simulink model "sistema_term"  (R2021b)
settings: Solver=FixedStepDiscrete  StartTime=0.0  StopTime=90  FixedStep=Tint  RelTol=1e-3
InitFcn:
  | init_fcn
values from neighbouring files (symbols this model uses):
  C_load = 5e-2    (= 0.05)    [init_fcn.m]
  C_V = c_v * ro_air * volume_room    (= 220.63309632)    [init_fcn.m]
  K_cond = Window_area * k_glass / esp    (= 158.4)    [init_fcn.m]
  L_s = 5e-3    (= 0.005)    [init_fcn.m]
  shift = (180/3)/360 * Ts    (= 8.33333333333e-05)    [init_fcn.m]
  T_ext = 15    [init_fcn.m]
  Tint = 5e-5    (= 5e-05)    [init_fcn.m]
  Ts = 0.0005    [init_fcn.m]
  V_H4 = 300    [init_fcn.m]
  V_source = 230 * sqrt(2)    [init_fcn.m]
undefined symbols (not defined in the file or in its folder): DiscIntNeverNeededParam
libraries: spsIGBTDiodeLib x5, spsSeriesRLCBranchLib x4, spsCurrentMeasurementLib x4, spsVoltageMeasurementLib x4, slpidlib x3, simulink x3, spsACVoltageSourceLib x1, spsDiodeLib x1, spsParallelRLCBranchLib x1, spspowerguiLib x1
settings Model: Creator=david  LastModifiedBy=david

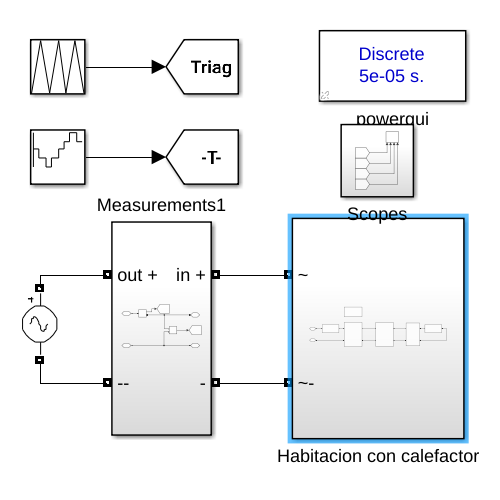
[thumbnail: Simulink's stored preview of the top-level diagram]
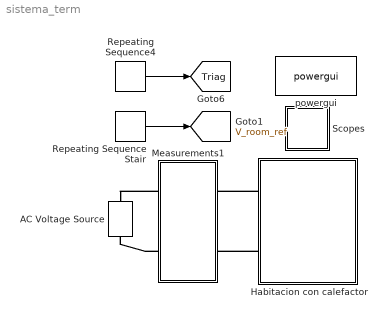
== system sistema_term ==
  AC Voltage Source : spsACVoltageSourceLib/AC Voltage Source  Amplitude=V_source  Phase=0  Frequency=50  SampleTime=0  Measurements=None  BusType=swing  Pref=10e3  Qref=0  Qmin=-inf  Qmax=+inf
  Habitacion con calefactor : Subsystem
  Measurements1 : Subsystem
  Repeating Sequence Stair : simulink/Sources/Repeating Sequence Stair  OutValues=[300 200 100 200 300 400 500 400].'  tsamp=10  OutMin=[]  OutMax=[]  OutDataTypeStr=double  OutputDataTypeScalingMode=double  OutDataType=fixdt(0,8)  ConRadixGroup=Best Precision: Vector-wise  OutScaling=2^-12
  Repeating Sequence4 : simulink/Sources/Repeating Sequence  rep_seq_t=[0 Ts/2 Ts]  rep_seq_y=[-1 1 -1]
  Scopes : Subsystem
  powergui : spspowerguiLib/powergui  Priority=1  SimulationMode=Discrete  SampleTime=Tint  frequency=60  Iterations=50  frequencyindice=0  Pbase=100e6  ErrMax=1e-4  UnitsV=kV  UnitsW=MW  buscounter=0  FunctionMessages=off  echomessages=off  EnableUseOfTLC=off  CurrentSourceSwitches=off  DisableSnubberDevices=off  DisableRonSwitches=off  DisableVfSwitches=off  DisplayEquations=off  AutomaticDiscreteSolvers=off  SolverType=Tustin/Backward Euler (TBE)  Interpol=off  ExternalGateDelay=off  methode=off  Ts=100  x0status=blocks  SPID=on  SwTol=0  HookPort=off  NonlinearTolerance=1e-4  nMaxIteration=100  ContinueOnMaxIteration=off  RestoreLinks=warning  ResistiveCurrentMeasurement=off  Frange=[0:2:500]  Ylog=off  Xlog=on  ShowGrid=off  save=off  variable=ZData  structure=0  ZoomFFT=off  StartTime=0.0  cycles=1  DisplayStyle=1  fundamental=60  FreqAxis=off  MaxFrequency=1000  frequencyindicesteady=1  RmsSteady=1  display=off
  tag scope: Triag=global, V_room_ref=global
  wires:
  Repeating Sequence4/1 -> [Triag]
  Repeating Sequence Stair/1 -> [V_room_ref]
  connections:
  Measurements1/RConn1 -- AC Voltage Source/RConn1
  Measurements1/RConn2 -- AC Voltage Source/LConn1
  Habitacion con calefactor/LConn1 -- Measurements1/LConn1
  Habitacion con calefactor/LConn2 -- Measurements1/LConn2

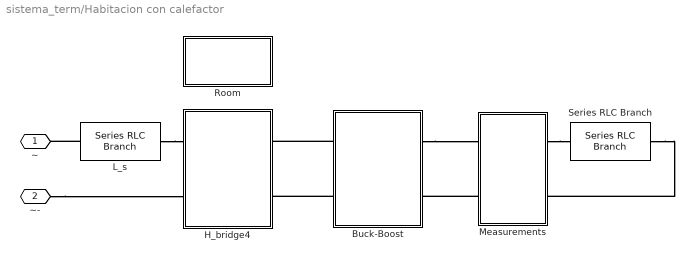
== system sistema_term/Habitacion con calefactor ==
  Buck-Boost : Subsystem
  H_bridge4 : Subsystem
  L_s : spsSeriesRLCBranchLib/Series RLC Branch  LConnTagsString=__new0  RConnTagsString=__new0  BranchType=L  Resistance=1  Inductance=L_s  SetiL0=off  InitialCurrent=0  Capacitance=1e-6  Setx0=off  InitialVoltage=0  Measurements=None
  Measurements : Subsystem
  Room : Subsystem
  Series RLC Branch : spsSeriesRLCBranchLib/Series RLC Branch  LConnTagsString=__new0  RConnTagsString=__new0  BranchType=R  Resistance=100  Inductance=1e-3  SetiL0=off  InitialCurrent=0  Capacitance=1e-6  Setx0=off  InitialVoltage=0  Measurements=None
  ~ : PMIOPort  Side=Left
  ~- : PMIOPort  Port=2  Side=Left
  connections:
  ~-/RConn1 -- H_bridge4/RConn2
  L_s/LConn1 -- H_bridge4/RConn1
  L_s/RConn1 -- ~/RConn1
  Measurements/RConn1 -- Series RLC Branch/LConn1
  Series RLC Branch/RConn1 -- Measurements/RConn2
  Buck-Boost/RConn1 -- Measurements/LConn1
  Measurements/LConn2 -- Buck-Boost/RConn2
  Buck-Boost/LConn2 -- H_bridge4/LConn2
  Buck-Boost/LConn1 -- H_bridge4/LConn1

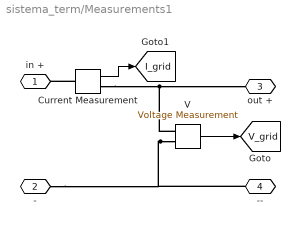
== system sistema_term/Measurements1 ==
  Current Measurement : spsCurrentMeasurementLib/Current Measurement  PhasorSimulation=off  OutputType=Complex  PSBequivalent=0
  V : spsVoltageMeasurementLib/Voltage Measurement  PhasorSimulation=off  OutputType=Complex  PSBequivalent=0
  in + : PMIOPort  Side=Left
  - : PMIOPort  Port=2  Side=Left
  out + : PMIOPort  Port=3  Side=Right
  -- : PMIOPort  Port=4  Side=Right
  tag scope: I_grid=global, V_grid=global
  wires:
  V/1 -> [V_grid]
  Current Measurement/1 -> [I_grid]
  connections:
  V/LConn2 -- --/RConn1 -- -/RConn1
  V/LConn1 -- Current Measurement/RConn1 -- out +/RConn1
  Current Measurement/LConn1 -- in +/RConn1

== system sistema_term/Scopes ==
  Scope : Scope  NumInputPorts=4
  wires:
  [V_room_ref] -> Scope/2
  [T_room] -> Scope/1
  [V_room] -> Scope/4
  [P_room] -> Scope/3

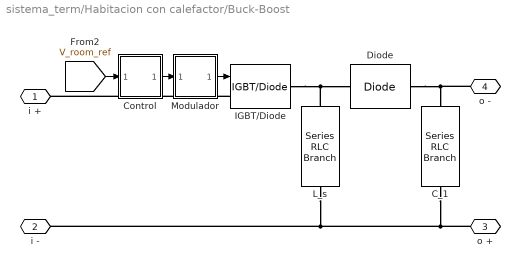
== system sistema_term/Habitacion con calefactor/Buck-Boost ==
  C_1 : spsSeriesRLCBranchLib/Series RLC Branch  LConnTagsString=__new0  RConnTagsString=__new0  BranchType=C  Resistance=1  Inductance=L_s/2  SetiL0=off  InitialCurrent=0  Capacitance=C_load/4  Setx0=on  InitialVoltage=300  Measurements=None
  Control : Subsystem
  Diode : spsDiodeLib/Diode  Ron=1e-3  Lon=0  Vf=0.8  IC=0  UseSnubber=0  Rs=1e3  Cs=250e-9  Measurements=off
  IGBT/Diode : spsIGBTDiodeLib/IGBT//Diode  Ron=1e-3  Rs=1e5  Cs=inf  Measurements=off
  L_s : spsSeriesRLCBranchLib/Series RLC Branch  LConnTagsString=__new0  RConnTagsString=__new0  BranchType=L  Resistance=1  Inductance=L_s * 12  SetiL0=off  InitialCurrent=0  Capacitance=1e-6  Setx0=off  InitialVoltage=0  Measurements=None
  Modulador : Subsystem
  i + : PMIOPort  Side=Left
  i - : PMIOPort  Port=2  Side=Left
  o + : PMIOPort  Port=3  Side=Right
  o - : PMIOPort  Port=4  Side=Right
  wires:
  Control/1(Out1) -> Modulador/1(In1)
  Modulador/1(Out1) -> IGBT/Diode/1
  [V_room_ref] -> Control/1(In1)
  connections:
  C_1/LConn1 -- L_s/LConn1 -- i -/RConn1 -- o +/RConn1
  L_s/RConn1 -- Diode/RConn1 -- IGBT/Diode/RConn1
  o -/RConn1 -- Diode/LConn1 -- C_1/RConn1
  IGBT/Diode/LConn1 -- i +/RConn1

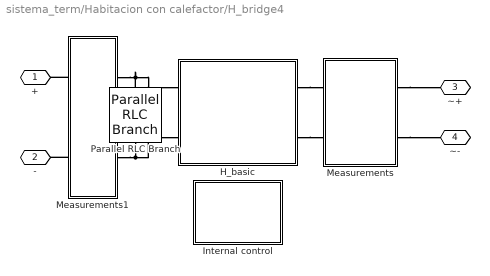
== system sistema_term/Habitacion con calefactor/H_bridge4 ==
  H_basic : Subsystem
  Internal control : Subsystem
  Measurements : Subsystem
  Measurements1 : Subsystem
  Parallel RLC Branch : spsParallelRLCBranchLib/Parallel RLC Branch  LConnTagsString=a  RConnTagsString=__new0  BranchType=C  Resistance=1  Inductance=1e-3  SetiL0=off  InitialCurrent=0  Capacitance=C_load  Setx0=on  InitialVoltage=C_init_v  Measurements=None
  + : PMIOPort  Side=Left
  - : PMIOPort  Port=2  Side=Left
  ~+ : PMIOPort  Port=3  Side=Right
  ~- : PMIOPort  Port=4  Side=Right
  connections:
  Measurements1/RConn1 -- Parallel RLC Branch/LConn1 -- H_basic/LConn1
  Measurements/LConn1 -- ~+/RConn1
  Measurements1/RConn2 -- Parallel RLC Branch/RConn1 -- H_basic/LConn2
  Measurements1/LConn1 -- +/RConn1
  Measurements1/LConn2 -- -/RConn1
  H_basic/RConn2 -- Measurements/RConn2
  Measurements/LConn2 -- ~-/RConn1
  H_basic/RConn1 -- Measurements/RConn1

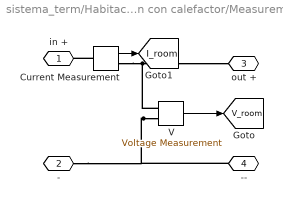
== system sistema_term/Habitacion con calefactor/Measurements ==
  Current Measurement : spsCurrentMeasurementLib/Current Measurement  PhasorSimulation=off  OutputType=Complex  PSBequivalent=0
  V : spsVoltageMeasurementLib/Voltage Measurement  PhasorSimulation=off  OutputType=Complex  PSBequivalent=0
  in + : PMIOPort  Side=Left
  - : PMIOPort  Port=2  Side=Left
  out + : PMIOPort  Port=3  Side=Right
  -- : PMIOPort  Port=4  Side=Right
  tag scope: I_room=global, V_room=global
  wires:
  V/1 -> [V_room]
  Current Measurement/1 -> [I_room]
  connections:
  V/LConn2 -- --/RConn1 -- -/RConn1
  V/LConn1 -- Current Measurement/RConn1 -- out +/RConn1
  Current Measurement/LConn1 -- in +/RConn1

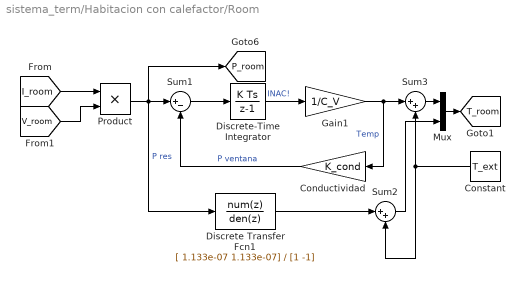
== system sistema_term/Habitacion con calefactor/Room ==
  Conductividad : Gain  Gain=K_cond
  Constant : Constant  Value=T_ext
  Discrete Transfer Fcn1 : DiscreteTransferFcn  Numerator=[ 1.133e-07 1.133e-07]  Denominator=[1 -1]  SampleTime=1
  Discrete-Time Integrator : DiscreteIntegrator  SampleTime=Tint  ICPrevOutput=DiscIntNeverNeededParam  ICPrevScaledInput=DiscIntNeverNeededParam
  Gain1 : Gain  Gain=1/C_V
  Mux : Mux  Inputs=2
  Product : Product
  Sum1 : Sum  Inputs=|+-
  Sum2 : Sum  Inputs=|++
  Sum3 : Sum  Inputs=|++
  tag scope: P_room=global, T_room=global
  wires:
  Sum1/1 -> Discrete-Time Integrator/1
  Discrete-Time Integrator/1 -> Gain1/1  "INAC!"
  Gain1/1 -> Conductividad/1, Sum3/1  "Temp"
  Conductividad/1 -> Sum1/2  "P ventana"
  [V_room] -> Product/2
  [I_room] -> Product/1
  Product/1 -> [P_room], Discrete Transfer Fcn1/1, Sum1/1  "P res"
  Constant/1 -> Sum3/2, Sum2/2
  Discrete Transfer Fcn1/1 -> Sum2/1
  Sum2/1 -> Mux/2
  Sum3/1 -> Mux/1
  Mux/1 -> [T_room]

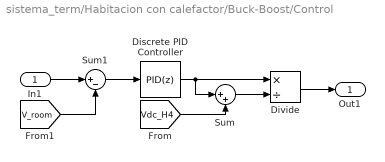
== system sistema_term/Habitacion con calefactor/Buck-Boost/Control ==
  In1 : Inport
  Discrete PID Controller : slpidlib/PID Controller  Controller=PID  Form=Parallel  TimeDomain=Discrete-time  UseExternalTs=off  SampleTime=Ts  IntegratorMethod=Forward Euler  FilterMethod=Forward Euler  ControllerParametersSource=internal  P=2  I=10  D=0.05  UseFilter=on  N=100  TunerSelectOption=Transfer Function Based (PID Tuner App)  InitialConditionSource=internal  InitialConditionForIntegrator=0  InitialConditionForFilter=0  DifferentiatorICPrevScaledInput=0  ExternalReset=none  TrackingMode=off  Kt=1  LimitOutput=off  SatLimitsSource=internal  UpperSaturationLimit=inf  LowerSaturationLimit=-inf  LinearizeAsGain=off  AntiWindupMode=none  Kb=1  POutMin=[]  POutMax=[]  IOutMin=[]  IOutMax=[]  DOutMin=[]  DOutMax=[]  NOutMin=[]  NOutMax=[]  SumOutMin=[]  SumOutMax=[]  SaturationOutMin=[]  SaturationOutMax=[]  PParamMin=[]  PParamMax=[]  IParamMin=[]  IParamMax=[]  DParamMin=[]  DParamMax=[]  NParamMin=[]  NParamMax=[]  KbParamMin=[]  KbParamMax=[]  KtParamMin=[]  KtParamMax=[]  KbOutMin=[]  KbOutMax=[]  KtOutMin=[]  KtOutMax=[]  IntegratorOutMin=[]  IntegratorOutMax=[]  FilterOutMin=[]  FilterOutMax=[]  SumI1OutMin=[]  SumI1OutMax=[]  SumI2OutMin=[]  SumI2OutMax=[]  SumI3OutMin=[]  SumI3OutMax=[]  SumI4OutMin=[]  SumI4OutMax=[]  SumDOutMin=[]  SumDOutMax=[]  DifferentiatorOutMin=[]  DifferentiatorOutMax=[]  FilterDiffOutCoefMin=[]  FilterDiffOutCoefMax=[]  ReciprocalOutMin=[]  ReciprocalOutMax=[]  SumDenOutMin=[]  SumDenOutMax=[]  SumNumOutMin=[]  SumNumOutMax=[]  DivideOutMin=[]  DivideOutMax=[]  UdiffTsProdOutMin=[]  UdiffTsProdOutMax=[]  NTsProdOutMin=[]  NTsProdOutMax=[]  UintegralTsProdOutMin=[]  UintegralTsProdOutMax=[]  UngainTsProdOutMin=[]  UngainTsProdOutMax=[]  IntegratorContinuousStateAttributes=''  IntegratorStateMustResolveToSignalObject=off  IntegratorRTWStateStorageClass=Auto  FilterContinuousStateAttributes=''  FilterStateMustResolveToSignalObject=off  FilterRTWStateStorageClass=Auto  ParallelPVariant=InternalParameters  IdealPVariant=Disabled  IVariant=InternalParameters  DVariant=InternalParameters  IntegratorVariant=Discrete  SatVariant=Disabled  AWVariant=Passthrough  PCopyVariant=Disabled  TRVariant=Disabled  FdbkBlocksVariant=Forward  IdealPFdbkVariant=Disabled  SatFdbkVariant=Disabled  DerivativeFilterVariant=ForwardEulerFilter  NVariant=InternalParameters  NCopyVariant=Disabled  FilterICVariant=InternalICsFilter  IntegratorICVariant=InternalICs  ExternalResetVariant=Disabled  TRSumVariant=Passthrough  SumFdbkVariant=Disabled  SumVariant=Sum_PID  TsampFilterVariant=InternalTs  TsampNgainVariant=Passthrough  TsampIntegralVariant=Passthrough  ExternalSaturationOutDataTypeStr=Inherit: Same as second input
  Divide : Product  Inputs=*/
  Sum : Sum  Inputs=|++
  Sum1 : Sum  Inputs=|+-
  Out1 : Outport
  wires:
  [V_room] -> Sum1/2
  In1/1 -> Sum1/1
  Divide/1 -> Out1/1
  [Vdc_H4] -> Sum/2
  Sum/1 -> Divide/2
  Discrete PID Controller/1 -> Divide/1, Sum/1
  Sum1/1 -> Discrete PID Controller/1

== system sistema_term/Habitacion con calefactor/Buck-Boost/Modulador ==
  In1 : Inport
  Relational Operator : RelationalOperator  OutDataTypeStr=boolean  RndMeth=Simplest
  Repeating Sequence4 : simulink/Sources/Repeating Sequence  rep_seq_t=[0 Ts/2 Ts]  rep_seq_y=[0 1 0]
  Out1 : Outport
  wires:
  In1/1 -> Relational Operator/1
  Relational Operator/1 -> Out1/1
  Repeating Sequence4/1 -> Relational Operator/2

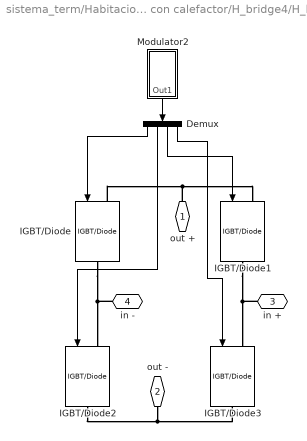
== system sistema_term/Habitacion con calefactor/H_bridge4/H_basic ==
  Demux : Demux
  IGBT/Diode{,1..3} (4 alike) : spsIGBTDiodeLib/IGBT//Diode  Ron=1e-3  Rs=1e5  Cs=inf  Measurements=off
  Modulator2 : Subsystem
  out + : PMIOPort  Side=Left
  out - : PMIOPort  Port=2  Side=Left
  in + : PMIOPort  Port=3  Side=Right
  in - : PMIOPort  Port=4  Side=Right
  wires:
  Demux/1 -> IGBT/Diode/1
  Demux/4 -> IGBT/Diode3/1
  Demux/2 -> IGBT/Diode2/1
  Demux/3 -> IGBT/Diode1/1
  Modulator2/1(Out1) -> Demux/1
  connections:
  IGBT/Diode2/RConn1 -- out -/RConn1 -- IGBT/Diode3/RConn1
  IGBT/Diode1/RConn1 -- in +/RConn1 -- IGBT/Diode3/LConn1
  IGBT/Diode/LConn1 -- out +/RConn1 -- IGBT/Diode1/LConn1
  IGBT/Diode/RConn1 -- in -/RConn1 -- IGBT/Diode2/LConn1

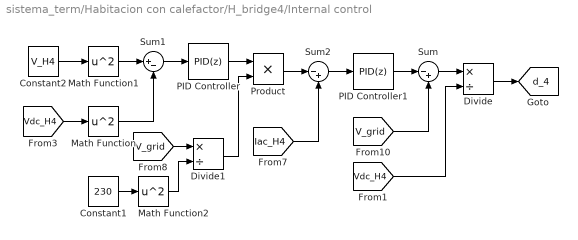
== system sistema_term/Habitacion con calefactor/H_bridge4/Internal control ==
  Constant1 : Constant  Value=230
  Constant2 : Constant  Value=V_H4
  Divide : Product  Inputs=*/
  Divide1 : Product  Inputs=*/
  Math Function : Math  Operator=square  SaturateOnIntegerOverflow=on
  Math Function1 : Math  Operator=square  SaturateOnIntegerOverflow=on
  Math Function2 : Math  Operator=square  SaturateOnIntegerOverflow=on
  PID Controller : slpidlib/PID Controller  Controller=PID  Form=Parallel  TimeDomain=Discrete-time  UseExternalTs=off  SampleTime=Ts  IntegratorMethod=Forward Euler  FilterMethod=Forward Euler  ControllerParametersSource=internal  P=2  I=10  D=0  UseFilter=on  N=100  TunerSelectOption=Transfer Function Based (PID Tuner App)  InitialConditionSource=internal  InitialConditionForIntegrator=0  InitialConditionForFilter=0  DifferentiatorICPrevScaledInput=0  ExternalReset=none  TrackingMode=off  Kt=1  LimitOutput=off  SatLimitsSource=internal  UpperSaturationLimit=inf  LowerSaturationLimit=-inf  LinearizeAsGain=on  AntiWindupMode=none  Kb=1  POutMin=[]  POutMax=[]  IOutMin=[]  IOutMax=[]  DOutMin=[]  DOutMax=[]  NOutMin=[]  NOutMax=[]  SumOutMin=[]  SumOutMax=[]  SaturationOutMin=[]  SaturationOutMax=[]  PParamMin=[]  PParamMax=[]  IParamMin=[]  IParamMax=[]  DParamMin=[]  DParamMax=[]  NParamMin=[]  NParamMax=[]  KbParamMin=[]  KbParamMax=[]  KtParamMin=[]  KtParamMax=[]  KbOutMin=[]  KbOutMax=[]  KtOutMin=[]  KtOutMax=[]  IntegratorOutMin=[]  IntegratorOutMax=[]  FilterOutMin=[]  FilterOutMax=[]  SumI1OutMin=[]  SumI1OutMax=[]  SumI2OutMin=[]  SumI2OutMax=[]  SumI3OutMin=[]  SumI3OutMax=[]  SumI4OutMin=[]  SumI4OutMax=[]  SumDOutMin=[]  SumDOutMax=[]  DifferentiatorOutMin=[]  DifferentiatorOutMax=[]  FilterDiffOutCoefMin=[]  FilterDiffOutCoefMax=[]  ReciprocalOutMin=[]  ReciprocalOutMax=[]  SumDenOutMin=[]  SumDenOutMax=[]  SumNumOutMin=[]  SumNumOutMax=[]  DivideOutMin=[]  DivideOutMax=[]  UdiffTsProdOutMin=[]  UdiffTsProdOutMax=[]  NTsProdOutMin=[]  NTsProdOutMax=[]  UintegralTsProdOutMin=[]  UintegralTsProdOutMax=[]  UngainTsProdOutMin=[]  UngainTsProdOutMax=[]  IntegratorContinuousStateAttributes=''  IntegratorStateMustResolveToSignalObject=off  IntegratorRTWStateStorageClass=Auto  FilterContinuousStateAttributes=''  FilterStateMustResolveToSignalObject=off  FilterRTWStateStorageClass=Auto  ParallelPVariant=InternalParameters  IdealPVariant=Disabled  IVariant=InternalParameters  DVariant=InternalParameters  IntegratorVariant=Discrete  SatVariant=Disabled  AWVariant=Passthrough  PCopyVariant=Disabled  TRVariant=Disabled  FdbkBlocksVariant=Forward  IdealPFdbkVariant=Disabled  SatFdbkVariant=Disabled  DerivativeFilterVariant=ForwardEulerFilter  NVariant=InternalParameters  NCopyVariant=Disabled  FilterICVariant=InternalICsFilter  IntegratorICVariant=InternalICs  ExternalResetVariant=Disabled  TRSumVariant=Passthrough  SumFdbkVariant=Disabled  SumVariant=Sum_PID  TsampFilterVariant=InternalTs  TsampNgainVariant=Passthrough  TsampIntegralVariant=Passthrough  ExternalSaturationOutDataTypeStr=Inherit: Same as second input
  PID Controller1 : slpidlib/PID Controller  Controller=PID  Form=Parallel  TimeDomain=Discrete-time  UseExternalTs=off  SampleTime=Ts  IntegratorMethod=Forward Euler  FilterMethod=Forward Euler  ControllerParametersSource=internal  P=5  I=10  D=0  UseFilter=on  N=100  TunerSelectOption=Transfer Function Based (PID Tuner App)  InitialConditionSource=internal  InitialConditionForIntegrator=0  InitialConditionForFilter=0  DifferentiatorICPrevScaledInput=0  ExternalReset=none  TrackingMode=off  Kt=1  LimitOutput=off  SatLimitsSource=internal  UpperSaturationLimit=inf  LowerSaturationLimit=-inf  LinearizeAsGain=on  AntiWindupMode=none  Kb=1  POutMin=[]  POutMax=[]  IOutMin=[]  IOutMax=[]  DOutMin=[]  DOutMax=[]  NOutMin=[]  NOutMax=[]  SumOutMin=[]  SumOutMax=[]  SaturationOutMin=[]  SaturationOutMax=[]  PParamMin=[]  PParamMax=[]  IParamMin=[]  IParamMax=[]  DParamMin=[]  DParamMax=[]  NParamMin=[]  NParamMax=[]  KbParamMin=[]  KbParamMax=[]  KtParamMin=[]  KtParamMax=[]  KbOutMin=[]  KbOutMax=[]  KtOutMin=[]  KtOutMax=[]  IntegratorOutMin=[]  IntegratorOutMax=[]  FilterOutMin=[]  FilterOutMax=[]  SumI1OutMin=[]  SumI1OutMax=[]  SumI2OutMin=[]  SumI2OutMax=[]  SumI3OutMin=[]  SumI3OutMax=[]  SumI4OutMin=[]  SumI4OutMax=[]  SumDOutMin=[]  SumDOutMax=[]  DifferentiatorOutMin=[]  DifferentiatorOutMax=[]  FilterDiffOutCoefMin=[]  FilterDiffOutCoefMax=[]  ReciprocalOutMin=[]  ReciprocalOutMax=[]  SumDenOutMin=[]  SumDenOutMax=[]  SumNumOutMin=[]  SumNumOutMax=[]  DivideOutMin=[]  DivideOutMax=[]  UdiffTsProdOutMin=[]  UdiffTsProdOutMax=[]  NTsProdOutMin=[]  NTsProdOutMax=[]  UintegralTsProdOutMin=[]  UintegralTsProdOutMax=[]  UngainTsProdOutMin=[]  UngainTsProdOutMax=[]  IntegratorContinuousStateAttributes=''  IntegratorStateMustResolveToSignalObject=off  IntegratorRTWStateStorageClass=Auto  FilterContinuousStateAttributes=''  FilterStateMustResolveToSignalObject=off  FilterRTWStateStorageClass=Auto  ParallelPVariant=InternalParameters  IdealPVariant=Disabled  IVariant=InternalParameters  DVariant=InternalParameters  IntegratorVariant=Discrete  SatVariant=Disabled  AWVariant=Passthrough  PCopyVariant=Disabled  TRVariant=Disabled  FdbkBlocksVariant=Forward  IdealPFdbkVariant=Disabled  SatFdbkVariant=Disabled  DerivativeFilterVariant=ForwardEulerFilter  NVariant=InternalParameters  NCopyVariant=Disabled  FilterICVariant=InternalICsFilter  IntegratorICVariant=InternalICs  ExternalResetVariant=Disabled  TRSumVariant=Passthrough  SumFdbkVariant=Disabled  SumVariant=Sum_PID  TsampFilterVariant=InternalTs  TsampNgainVariant=Passthrough  TsampIntegralVariant=Passthrough  ExternalSaturationOutDataTypeStr=Inherit: Same as second input
  Product : Product
  Sum : Sum  Inputs=|-+
  Sum1 : Sum  Inputs=|+-
  Sum2 : Sum  Inputs=|-+
  tag scope: d_4=global
  wires:
  Divide/1 -> [d_4]
  Math Function1/1 -> Sum1/1
  [Iac_H4] -> Sum2/2
  Sum1/1 -> PID Controller/1
  Math Function/1 -> Sum1/2
  PID Controller1/1 -> Sum/1
  [Vdc_H4] -> Math Function/1
  PID Controller/1 -> Product/1
  Divide1/1 -> Product/2
  [V_grid] -> Sum/2
  Sum2/1 -> PID Controller1/1
  Sum/1 -> Divide/1
  [Vdc_H4] -> Divide/2
  Constant1/1 -> Math Function2/1
  [V_grid] -> Divide1/1
  Math Function2/1 -> Divide1/2
  Product/1 -> Sum2/1
  Constant2/1 -> Math Function1/1

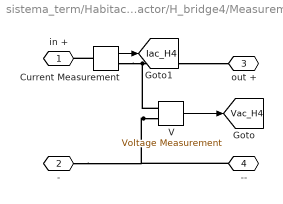
== system sistema_term/Habitacion con calefactor/H_bridge4/Measurements ==
  Current Measurement : spsCurrentMeasurementLib/Current Measurement  PhasorSimulation=off  OutputType=Complex  PSBequivalent=0
  V : spsVoltageMeasurementLib/Voltage Measurement  PhasorSimulation=off  OutputType=Complex  PSBequivalent=0
  in + : PMIOPort  Side=Left
  - : PMIOPort  Port=2  Side=Left
  out + : PMIOPort  Port=3  Side=Right
  -- : PMIOPort  Port=4  Side=Right
  tag scope: Iac_H4=global, Vac_H4=global
  wires:
  V/1 -> [Vac_H4]
  Current Measurement/1 -> [Iac_H4]
  connections:
  V/LConn2 -- --/RConn1 -- -/RConn1
  V/LConn1 -- Current Measurement/RConn1 -- out +/RConn1
  Current Measurement/LConn1 -- in +/RConn1

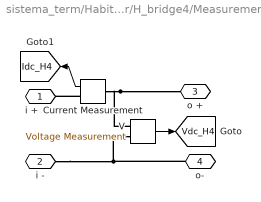
== system sistema_term/Habitacion con calefactor/H_bridge4/Measurements1 ==
  Current Measurement : spsCurrentMeasurementLib/Current Measurement  PhasorSimulation=off  OutputType=Complex  PSBequivalent=0
  V : spsVoltageMeasurementLib/Voltage Measurement  PhasorSimulation=off  OutputType=Complex  PSBequivalent=0
  i + : PMIOPort  Side=Left
  i - : PMIOPort  Port=2  Side=Left
  o + : PMIOPort  Port=3  Side=Right
  o- : PMIOPort  Port=4  Side=Right
  tag scope: Idc_H4=global, Vdc_H4=global
  wires:
  V/1 -> [Vdc_H4]
  Current Measurement/1 -> [Idc_H4]
  connections:
  i -/RConn1 -- V/LConn2 -- o-/RConn1
  V/LConn1 -- Current Measurement/LConn1 -- o +/RConn1
  Current Measurement/RConn1 -- i +/RConn1

== system sistema_term/Habitacion con calefactor/H_bridge4/H_basic/Modulator2 ==
  Mux : Mux
  Restriccion : Subsystem
  Transport Delay : TransportDelay  DelayTime=shift
  Unipolar : Subsystem
  Out1 : Outport
  wires:
  Restriccion/1(Out1) -> Mux/1
  [d_4] -> Unipolar/1(Duty)
  Mux/1 -> Out1/1
  Restriccion/4(Out4) -> Mux/4
  Unipolar/1(Out1) -> Restriccion/1(In1)
  Restriccion/3(Out3) -> Mux/3
  Unipolar/2(Out2) -> Restriccion/2(In2)
  Restriccion/2(Out2) -> Mux/2
  [Triag] -> Transport Delay/1
  Transport Delay/1 -> Unipolar/2(Triag)

== system sistema_term/Habitacion con calefactor/H_bridge4/H_basic/Modulator2/Restriccion ==
  In1 : Inport
  In2 : Inport  Port=2
  Logical Operator1 : Logic  Operator=NOT  AllPortsSameDT=off  OutDataTypeStr=boolean
  Logical Operator2 : Logic  Operator=NOT  AllPortsSameDT=off  OutDataTypeStr=boolean
  Out1 : Outport
  Out2 : Outport  Port=2
  Out3 : Outport  Port=3
  Out4 : Outport  Port=4
  wires:
  In1/1 -> Out1/1, Logical Operator1/1
  In2/1 -> Out3/1, Logical Operator2/1
  Logical Operator2/1 -> Out4/1
  Logical Operator1/1 -> Out2/1

== system sistema_term/Habitacion con calefactor/H_bridge4/H_basic/Modulator2/Unipolar ==
  Duty : Inport
  Triag : Inport  Port=2
  Gain : Gain  Gain=-1
  Relational Operator : RelationalOperator  OutDataTypeStr=boolean  RndMeth=Simplest
  Relational Operator1 : RelationalOperator  OutDataTypeStr=boolean  RndMeth=Simplest
  Out1 : Outport
  Out2 : Outport  Port=2
  wires:
  Relational Operator/1 -> Out1/1
  Triag/1 -> Relational Operator/2, Gain/1
  Duty/1 -> Relational Operator1/2, Relational Operator/1
  Relational Operator1/1 -> Out2/1
  Gain/1 -> Relational Operator1/1
